simulink subsystem "Acondicionamiento_Sensor_laser"  (R2023b)
settings: Solver=VariableStepAuto  StartTime=0.0  StopTime=10.0  RelTol=1e-3
settings Model: Creator=manu_  LastModifiedBy=manu_

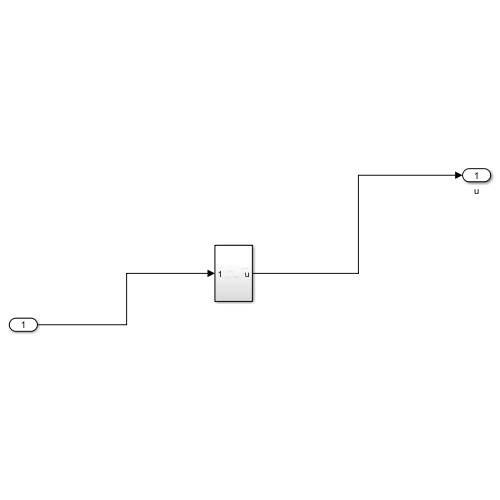
[thumbnail: Simulink's stored preview of the top-level diagram]
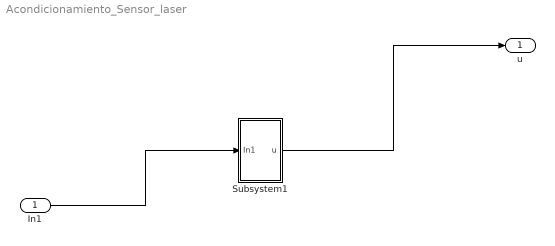
== system Acondicionamiento_Sensor_laser ==
  In1 : Inport
  Subsystem1 : Subsystem
  u : Outport
  wires:
  Subsystem1/1(u) -> u/1
  In1/1 -> Subsystem1/1(In1)

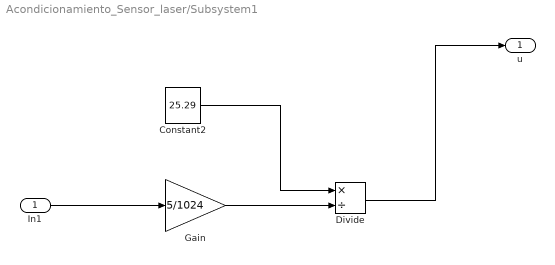
== system Acondicionamiento_Sensor_laser/Subsystem1 ==
  In1 : Inport
  Constant2 : Constant  Value=25.29
  Divide : Product  Inputs=*/
  Gain : Gain  Gain=5/1024
  u : Outport
  wires:
  Constant2/1 -> Divide/1
  In1/1 -> Gain/1
  Gain/1 -> Divide/2
  Divide/1 -> u/1
